simulink model "t4_ejercicio1"  (R2024a)
settings: Solver=ode1  StartTime=0.0  StopTime=300  FixedStep=0.01  MaxStep=1e-2  RelTol=1e-5
settings Model: Creator=pablo  LastModifiedBy=pablo

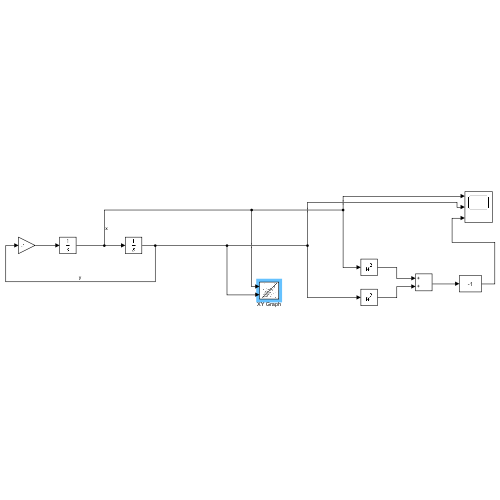
[thumbnail: Simulink's stored preview of the top-level diagram]
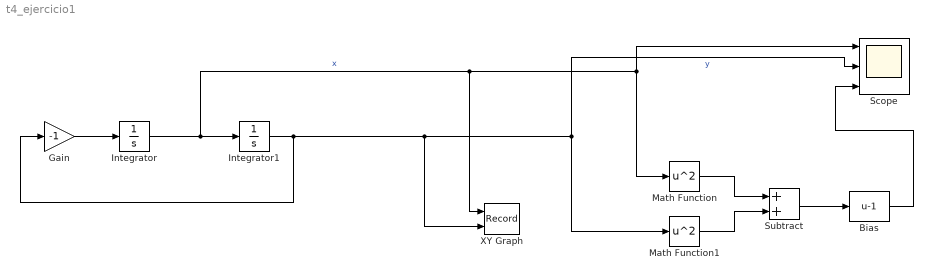
== system t4_ejercicio1 ==
  Bias : Bias  Bias=-1  SaturateOnIntegerOverflow=off
  Gain : Gain  Gain=-1
  Integrator : Integrator  InitialCondition=1
  Integrator1 : Integrator
  Math Function : Math  Operator=square
  Math Function1 : Math  Operator=square
  Scope : Scope  NumInputPorts=3
  Subtract : Sum
  XY Graph : Record  FileSettingsInternal="{\"entries\":[{\"content\":{\"excelSettings\":{\"content\":{},\"type\":\"Streamout.ExcelSettings\"}},\"type\":\"Streamout.FileSettingStorage\",\"uuid\":\"\"}],\"packageUris\":[\"http:\\/\\/schema.mathworks.com\\/mf0\\/streamout_blocks\\/R2020a\"],\"version\":\"1.0\"}"  Layout=[1 1]  SignalsInternal="{\"entries\":[{\"content\":{\"signals\":[{\"content\":{\"blockPath\":[],\"dimensions\":[1],\"domain\":\"\",\"lineColor\":\"#a2142f\",\"plots\":[ 1 ],\"port\":1,\"sid\":[\"\"],\"signalID\":1,\"signalName\":\"x\"},\"type\":\"RecordBlkView.Signal\",\"uuid\":\"\"},{\"content\":{\"blockPath\":[],\"dimensions\":[1],\"domain\":\"\",\"lineColor\":\"#139fff\",\"plots\":[ 1 ],\"port\":2,\"sid\":[\"\"],\"signalID\":2,\"signalName\":\"y\"},\"type\":\"RecordBlkView.Signal\",\"uuid\":\"\"}]},\"type\":\"RecordBlkView.InputSignals\",\"uuid\":\"\"}],\"packageUris\":[\"http:\\/\\/schema.mathworks.com\\/mf0\\/streamout_blocks\\/R2020a\"],\"version\":\"1.0\"}"  VisualizationBindings="{\"xyplotplugin\":{\"info\":[{\"series\":[{\"bindingParametersList\":[{\"parameter\":\"X-Axis\",\"signalID\":1,\"signalName\":\"x\"},{\"parameter\":\"Y-Axis\",\"signalID\":2,\"signalName\":\"y\"}],\"seriesID\":0}],\"subplotID\":1}]}}"  CompatibilityTag=XY
  wires:
  Integrator/1 -> XY Graph/1, Math Function/1, Scope/1, Integrator1/1  "x"
  Integrator1/1 -> Gain/1, XY Graph/2, Math Function1/1, Scope/2  "y"
  Gain/1 -> Integrator/1
  Math Function/1 -> Subtract/1
  Math Function1/1 -> Subtract/2
  Subtract/1 -> Bias/1
  Bias/1 -> Scope/3
